simulink subsystem "System_complete"  (R2022a)
settings: Solver=VariableStepAuto  StartTime=0.0  StopTime=10.0  RelTol=1e-3
settings Model: Creator=Haier  LastModifiedBy=Haier

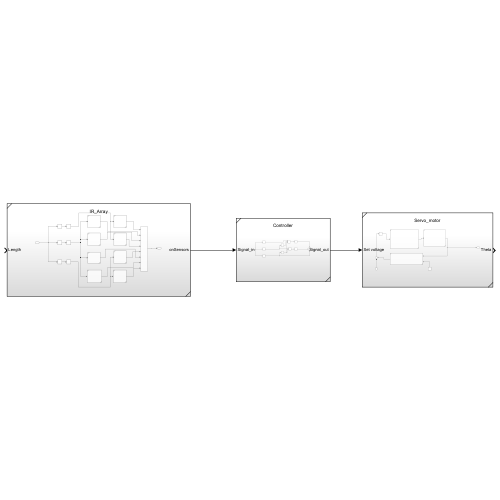
[thumbnail: Simulink's stored preview of the top-level diagram]
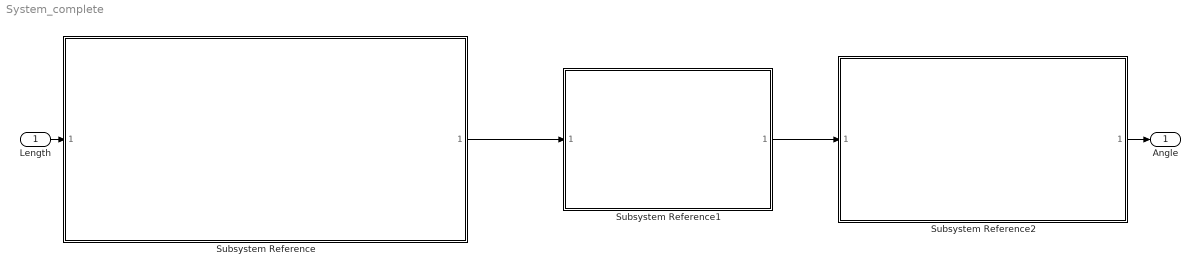
== system System_complete ==
  Length : Inport
  Subsystem Reference : Subsystem  ReferencedSubsystem=IR_Array
  Subsystem Reference1 : Subsystem  ReferencedSubsystem=Controller
  Subsystem Reference2 : Subsystem  ReferencedSubsystem=Servo_motor
  Angle : Outport
  wires:
  Subsystem Reference/1 -> Subsystem Reference1/1
  Subsystem Reference1/1 -> Subsystem Reference2/1
  Length/1 -> Subsystem Reference/1
  Subsystem Reference2/1 -> Angle/1
